simulink model "idontKnow2013a"  (R2013a)
settings: Solver=ode45  SolverMode=SingleTasking  StartTime=0.0  StopTime=500  MaxStep=1E-3  RelTol=1e-3
values from neighbouring files (symbols this model uses):
  A = [0,1;0,0]    [AAAA_trying.m]    (also in MPCController.m = plant.A; MPCController1.m; aaass.m; app1.m = 1)
  B = plant.B    [MPCController.m]    (also in MPCController1.m = [0,0;1,-1]; aaass.m = [b,-b])
  b = [0;1]    [AAAA_trying.m]    (also in aaass.m)
  C = plant.C    [MPCController.m]    (also in MPCController1.m = eye(2); aaass.m = eye(2))
  D = zeros(2,2)    [MPCController1.m]    (also in aaass.m)
  kd = 0.7021    [aaass.m]
  kp = 0.1859    [aaass.m]
  V = 1./(cT*inv(eye*(2) - Ad+bd*kT)*bd)    [aaass.m]
undefined symbols (not defined in the file or in its folder): K
libraries: simulink x1
settings Model: CovMetricSettings=dwe  CovHtmlReporting=off  covSaveCumulativeToWorkspaceVar=off  CovSaveSingleToWorkspaceVar=off  CovExternalEMLEnable=on  Creator=HP  LastModifiedBy=HP
settings DataIOCC: LimitDataPoints=off  SaveFormat=StructureWithTime
settings DebuggingCC: UnderspecifiedInitializationDetection=Simplified  MergeDetectMultiDrivingBlocksExec=error  SolverPrmCheckMsg=none  FrameProcessingCompatibilityMsg=error  StateNameClashWarn=none  SFUnexpectedBacktrackingDiag=error  SFNoUnconditionalDefaultTransitionDiag=error
settings HardwareCC: ProdBitPerPointer=64  ProdLargestAtomicFloat=Float  ProdIntDivRoundTo=Zero  ProdEndianess=LittleEndian  ProdHWDeviceType=Specified
settings ModelReferenceCC: PropagateSignalLabelsOutOfModel=on
settings SFSimCC: SimUseLocalCustomCode=on
settings RTWCC: RTWUseLocalCustomCode=on
settings GRTTargetCC: CodeReplacementLibrary=C99 (ISO)  GeneratePreprocessorConditionals=Use local settings

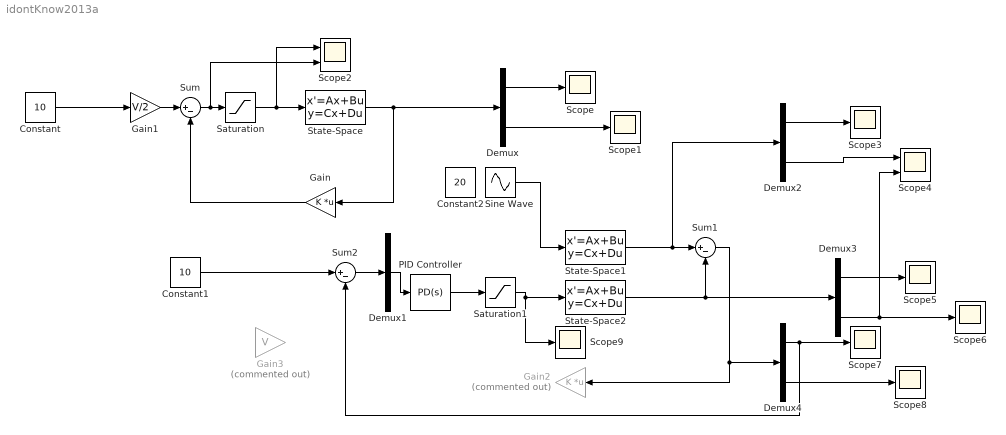
== system idontKnow2013a ==
  Constant : Constant  Value=10
  Constant1 : Constant  Value=10
  Constant2 : Constant  Value=20
  Demux{,2..4} (4 alike) : Demux  Outputs=2
  Demux1 : Demux  Outputs=1
  Gain : Gain  Gain=K  Multiplication=Matrix(K*u)
  Gain1 : Gain  Gain=V/2
  Gain2 : Gain  Commented=on  Gain=K  Multiplication=Matrix(K*u)
  Gain3 : Gain  Commented=on  Gain=V
  PID Controller : simulink/Continuous/PID Controller  Controller=PD  Form=Parallel  TimeDomain=Continuous-time  SampleTime=-1  IntegratorMethod=Forward Euler  FilterMethod=Forward Euler  ControllerParametersSource=internal  P=-kp  I=1  D=-kd  UseFilter=on  N=100  InitialConditionSource=internal  InitialConditionForIntegrator=0  InitialConditionForFilter=0  DifferentiatorICPrevScaledInput=0  ExternalReset=none  TrackingMode=off  Kt=1  LimitOutput=off  UpperSaturationLimit=inf  LowerSaturationLimit=-inf  LinearizeAsGain=on  AntiWindupMode=none  Kb=1  POutMin=[]  POutMax=[]  IOutMin=[]  IOutMax=[]  DOutMin=[]  DOutMax=[]  NOutMin=[]  NOutMax=[]  SumOutMin=[]  SumOutMax=[]  SaturationOutMin=[]  SaturationOutMax=[]  PParamMin=[]  PParamMax=[]  IParamMin=[]  IParamMax=[]  DParamMin=[]  DParamMax=[]  NParamMin=[]  NParamMax=[]  KbParamMin=[]  KbParamMax=[]  KtParamMin=[]  KtParamMax=[]  KbOutMin=[]  KbOutMax=[]  KtOutMin=[]  KtOutMax=[]  IntegratorOutMin=[]  IntegratorOutMax=[]  FilterOutMin=[]  FilterOutMax=[]  SumI1OutMin=[]  SumI1OutMax=[]  SumI2OutMin=[]  SumI2OutMax=[]  SumI3OutMin=[]  SumI3OutMax=[]  SumDOutMin=[]  SumDOutMax=[]  DifferentiatorOutMin=[]  DifferentiatorOutMax=[]  IntegratorContinuousStateAttributes=''  IntegratorStateMustResolveToSignalObject=off  IntegratorRTWStateStorageClass=Auto  FilterContinuousStateAttributes=''  FilterStateMustResolveToSignalObject=off  FilterRTWStateStorageClass=Auto
  Saturation : Saturate  UpperLimit=5  LowerLimit=-8
  Saturation1 : Saturate  UpperLimit=5  LowerLimit=-8
  Scope{,1,3,5..9} (8 alike) : Scope
      Scope settings: TimeRange=auto  MaxDataPoints=5000  SaveToWorkspace=off  SaveName=ScopeData  YMin=-57.8667  YMax=17.83102  SampleTime=-1
      Scope1 settings: TimeRange=auto  MaxDataPoints=5000  SaveToWorkspace=off  YMin=-4.0058  YMax=16.05216  SampleTime=-1
      Scope3 settings: TimeRange=auto  MaxDataPoints=5000  SaveToWorkspace=off  YMin=-379.07205  YMax=3411.64848  SampleTime=-1
      Scope5 settings: TimeRange=auto  MaxDataPoints=5000  SaveToWorkspace=off  SaveName=ScopeData3  YMin=-490.38884  YMax=3413.49952  SampleTime=-1
      Scope6 settings: TimeRange=auto  MaxDataPoints=5000  SaveToWorkspace=off  SaveName=ScopeData4  YMin=-880.00000  YMax=120.00000  SampleTime=-1
      Scope7 settings: TimeRange=auto  MaxDataPoints=5000  SaveToWorkspace=off  SaveName=ScopeData5  YMin=-3.35772  YMax=111.48419  SampleTime=-1
      Scope8 settings: TimeRange=auto  MaxDataPoints=5000  SaveToWorkspace=off  SaveName=ScopeData6  YMin=-47.26571  YMax=56.7573  SampleTime=-1
      Scope9 settings: TimeRange=auto  MaxDataPoints=5000  SaveToWorkspace=off  SaveName=ScopeData7  YMin=-4.415  YMax=6.04611  SampleTime=-1
  Scope2 : Scope  NumInputPorts=2
      settings: TimeRange=auto  MaxDataPoints=5000  SaveToWorkspace=off  SaveName=ScopeData2  YMin=-1.1269~-5  YMax=8.16761~5  SampleTime=-1
  Scope4 : Scope  NumInputPorts=2
      settings: TimeRange=auto  MaxDataPoints=5000  SaveToWorkspace=off  SaveName=ScopeData2  YMin=17.91137~-5  YMax=38.7948~5  SampleTime=-1
  Sine Wave : Sin  SampleTime=0
  State-Space : StateSpace  A=A  B=B  C=C  D=D  X0=[-50;-2]
  State-Space1 : StateSpace  A=A  B=b  C=eye(2)  D=zeros(2,1)  X0=[0;20]
  State-Space2 : StateSpace  A=A  B=b  C=eye(2)  D=zeros(2,1)  X0=[-100;20]
  Sum : Sum  Inputs=|+-
  Sum1 : Sum  Inputs=|+-
  Sum2 : Sum  Inputs=|+-
  wires:
  State-Space/1 -> Demux/1, Gain/1
  Sum/1 -> Scope2/2, Saturation/1
  Gain/1 -> Sum/2
  Gain1/1 -> Sum/1
  Constant/1 -> Gain1/1
  Demux/1 -> Scope/1
  Demux/2 -> Scope1/1
  Saturation/1 -> Scope2/1, State-Space/1
  State-Space1/1 -> Demux2/1, Sum1/1
  State-Space2/1 -> Demux3/1, Sum1/2
  Sum1/1 -> Gain2/1, Demux4/1
  Sum2/1 -> Demux1/1
  Demux1/1 -> PID Controller/1
  Demux2/1 -> Scope3/1
  Demux2/2 -> Scope4/1
  Demux3/2 -> Scope4/2, Scope6/1
  Demux3/1 -> Scope5/1
  Demux4/1 -> Scope7/1, Sum2/2
  Demux4/2 -> Scope8/1
  Saturation1/1 -> Scope9/1, State-Space2/1
  Constant1/1 -> Sum2/1
  Sine Wave/1 -> State-Space1/1
  PID Controller/1 -> Saturation1/1
